simulink library "dspmathops"  (Simulink 6.0)
settings: Solver=ode45  SolverMode=SingleTasking  StartTime=0.0  StopTime=10.0  RelTol=1e-3
values from neighbouring files (symbols this model uses):
  D = D + B    [rebuffer_delay.m]
undefined symbols (not defined in the file or in its folder): dBval, fuzz_val, magnitude
libraries: dspsigattribs x2
settings Model: RequirementInfo=9  CovMetricSettings=d  ForwardingTableString=||__slOldName__||dspmathops/DSP Sum||__slNewName__||dspobslib/DSP Sum||__slOldName__||dspmathops/DSP Product||__slNewName__||dspobslib/DSP Product||__slOldName__||dspmathops/DSP Gain||__slNewName__||dspobslib/DSP Gain  Creator=don  LastModifiedBy=mlongfri  ExtModeAutoUpdateStatusClock=off  ProdHWDeviceType=Specified
settings DataIOCC: SignalLoggingName=logsOut
settings OptimizationCC: BooleanDataType=off
settings DebuggingCC: CheckExecutionContextPreStartOutputMsg=on  CheckExecutionContextRuntimeOutputMsg=on  SolverPrmCheckMsg=none
settings HardwareCC: ProdHWDeviceType=Specified  TargetUnknown=on
settings SFSimCC: SFSimApplyToAllLibs=on  SFSimBuildMode=Incremental

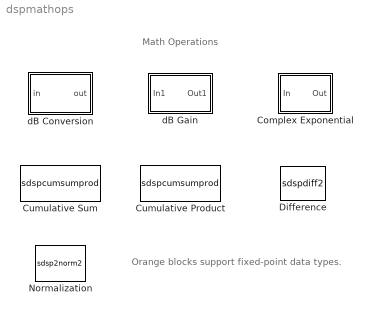
== system dspmathops ==
  note: Math Operations
  note: Orange blocks support fixed-point data types.
  Complex Exponential : Subsystem  PropExecContextAcrossSSBoundary=on
      mask Type: Complex Exponential
      mask Description:
      | Compute the complex exponential function of real inputs via
      | Euler's formula, y = cos(x)+jsin(x).
      mask Help: web(dspbhelp);
      mask Display: text(0.2, 0.55,'exp(jx)');
  Cumulative Product : S-Function  DialogController=dspDDGCreate  DialogControllerArgs=DataTag0  FunctionName=sdspcumsumprod  Parameters=dim,reset,fcn,dtInfo.interProdMode,dtInfo.interProdWordLength,dtInfo.interProdFracLength,dtInfo.prodOutputMode,dtInfo.prodOutputWordLength,dtInfo.prodOutputFracLength,dtInfo.accumMode,dtInfo.accumWordLength,dtInfo.accumFracLength,dtInfo.outputMode,dtInfo.outputWordLength,dtInfo.outputFracLength,dtInfo.roundingMode,dtInfo.overflowMode  mask(Cumulative Product){dim=Channels (running product), reset_popup=None, interProdMode=Same as input, interProdWordLength=16, interProdFracLength=15, prodOutputMode=Same as input, prodOutputWordLength=32, prodOutputFracLength=30, accumMode=Same as input, accumWordLength=32, accumFracLength=30, outputMode=Same as input, outputWordLength=16, outputFracLength=15, roundingMode=Floor, overflowMode=off, LockScale=off}
      mask prompts: dim "Multiply input along:"; reset_popup "Reset port:"; interProdMode "inter prod mode"; interProdWordLength "inter prod wl"; interProdFracLength "inter prod fl"; prodOutputMode "prod output mode"; prodOutputWordLength "prod output wl"; prodOutputFracLength "prod output fl"; accumMode "accum mode"; accumWordLength "accum wl"; accumFracLength "accum fl"; outputMode "output mode"; outputWordLength "output wl"; outputFracLength "output fl"; roundingMode "rm"; overflowMode "om"; LockScale "Lock scaling"
      mask help: Cumulative product of input matrix or input vector elements along the specified dimension: rows, columns, or channels. For 1-D and sample-based inputs, each element of the input matrix or vector is a channel. For frame-based inputs, each column of the input matrix or vector is a channel.
      mask init:
      | s = dspblkcumsumprod('icon');
      | reset=reset_popup-1;
      | fcn=1;
      | 
      | dtInfo = dspGetFixptDataTypeInfo(gcbh,271);
      settings: CopyFcn=dspfixptcopycallback
      mask Help: web(dspbhelp);
      mask StyleString: popup(Columns|Rows|Channels (running product)),popup(None|Rising edge|Falling edge|Either edge|Non-zero sample),popup(Same as input|Binary point scaling|Slope and bias scaling),edit,edit,popup(Same as input|Binary point scaling|Slope and bias scaling),edit,edit,popup(Same as product output|Same as input|Binary point scaling|Slope and bias scaling),edit,edit,popup(Same as product output|Same as input|Binary point scaling|Slope and bias scaling),edit,edit,popup(Floor|Nearest),checkbox,checkbox
      mask Display:
      | disp([s.str '\nProduct'])
      | port_label('input',s.i1,s.i1s);
      | port_label('input',s.i2,s.i2s);
  Cumulative Sum : S-Function  DialogController=dspDDGCreate  DialogControllerArgs=DataTag1  FunctionName=sdspcumsumprod  Parameters=dim,reset,fcn,-1,0,0,-1,0,0,dtInfo.accumMode,dtInfo.accumWordLength,dtInfo.accumFracLength,dtInfo.outputMode,dtInfo.outputWordLength,dtInfo.outputFracLength,dtInfo.roundingMode,dtInfo.overflowMode  mask(Cumulative Sum){dim=Channels (running sum), reset_popup=None, accumMode=Same as input, accumWordLength=32, accumFracLength=30, outputMode=Same as accumulator, outputWordLength=16, outputFracLength=15, roundingMode=Floor, overflowMode=off, LockScale=off}
      mask prompts: dim "Sum input along:"; reset_popup "Reset port:"; accumMode "accMode"; accumWordLength "accWL"; accumFracLength "accFL"; outputWordLength "outputWL"; outputFracLength "outputFL"; roundingMode "rm"; overflowMode "om"; LockScale "Lock scaling"
      mask help: Cumulative sum of input matrix or input vector elements along the specified dimension: rows, columns, or channels. For 1-D and sample-based inputs, each element of the input matrix or vector is a channel. For frame-based inputs, each column of the input matrix or vector is a channel.
      mask init:
      | s = dspblkcumsumprod('icon');
      | reset=reset_popup-1;
      | fcn=0;
      | 
      | dtInfo = dspGetFixptDataTypeInfo(gcbh,7);
      settings: CopyFcn=dspfixptcopycallback
      mask Help: web(dspbhelp);
      mask StyleString: popup(Columns|Rows|Channels (running sum)),popup(None|Rising edge|Falling edge|Either edge|Non-zero sample),popup(Same as input|Binary point scaling|Slope and bias scaling),edit,edit,popup(Same as accumulator|Same as input|Binary point scaling|Slope and bias scaling),edit,edit,popup(Floor|Nearest),checkbox,checkbox
      mask Display:
      | disp([s.str '\nSum'])
      | port_label('input',s.i1,s.i1s);
      | port_label('input',s.i2,s.i2s);
  Difference : S-Function  DialogController=dspDDGCreate  DialogControllerArgs=DataTag2  FunctionName=sdspdiff2  Parameters=dim,dtInfo.accumMode,dtInfo.accumWordLength,dtInfo.accumFracLength,dtInfo.outputMode,dtInfo.outputWordLength,dtInfo.outputFracLength,dtInfo.roundingMode,dtInfo.overflowMode  mask(Difference){dim=Columns, additionalParams=off, allowOverrides=on, outputMode=Same as accumulator, outputWordLength=16, outputFracLength=15, accumMode=Inherit via internal rule, accumWordLength=32, accumFracLength=30, roundingMode=Floor, overflowMode=off, LockScale=off}
      mask prompts: dim "Difference along:"; additionalParams "------- Show additional parameters -------"; allowOverrides "Allow overrides from DSP Fixed-Point Attributes blocks"; outputMode "Fixed-point output attributes:"; outputWordLength "Output word length:"; outputFracLength "Output fraction length:"; accumMode "Fixed-point accumulator attributes:"; accumWordLength "Accumulator word length:"; accumFracLength "Accumulator fraction length:"; roundingMode "Round integer calculations toward:"; overflowMode "Saturate on integer overflow"; LockScale "Lock scaling"
      mask help: Difference between adjacent input elements. For oriented inputs, difference along the specified dimension.
      mask init:
      | if (dim==1), str='Row\nDiff';
      | else str='Column\nDiff';
      | end
      | dtInfo = dspGetFixptDataTypeInfo(gcbh,7);
      settings: CopyFcn=dspfixptcopycallback
      mask Help: web(dspbhelp);
      mask StyleString: popup(Rows|Columns),checkbox,checkbox,popup(Same as accumulator|Same as input|Binary point scaling|Slope and bias scaling|User-defined),edit,edit,popup(Inherit via internal rule|Same as input|Binary point scaling|Slope and bias scaling|User-defined),edit,edit,popup(Floor|Nearest),checkbox,checkbox
      mask Display: disp(str)
  Normalization : S-Function  DialogController=dspDDGCreate  DialogControllerArgs=DataTag3  FunctionName=sdsp2norm2  Parameters=Bias,NormType,dtInfo.prodOutputMode,dtInfo.prodOutputWordLength,dtInfo.prodOutputFracLength,dtInfo.accumMode,dtInfo.accumWordLength,dtInfo.accumFracLength,dtInfo.outputMode,dtInfo.outputWordLength,dtInfo.outputFracLength,dtInfo.roundingMode,dtInfo.overflowMode  mask(Normalization){NormType=Squared 2-norm, Bias=1e-10, additionalParams=off, allowOverrides=on, outputMode=Same as product output, outputWordLength=32, outputFracLength=32, accumMode=Same as product output, accumWordLength=32, accumFracLength=30, prodOutputMode=Same as input, prodOutputWordLength=32, prodOutputFracLength=32, roundingMode=Floor, overflowMode=off, LockScale=off}
      mask prompts: NormType "Norm:"; Bias "Normalization bias:"; additionalParams "--------------- Show additional parameters ---------------"; allowOverrides "Allow overrides from DSP Attributes blocks"; outputMode "Fixed-point output attributes:"; outputWordLength "Output word length:"; outputFracLength "Output fraction length:"; accumMode "Fixed-point accumulator attributes"; accumWordLength "Accumulator word length:"; accumFracLength "Accumulator fraction length:"; prodOutputMode "Fixed-point product output attributes:"; prodOutputWordLength "Product output word length:"; prodOutputFracLength "Product output fraction length:"; roundingMode "Round integer calculations toward:"; overflowMode "Saturate on integer overflow"; LockScale "Lock scaling"
      mask help: Normalize each input element by the vector 2-norm, sqrt(u'u)+b, or by the squared 2-norm, u'u+b, where b is a bias used to protect against divide-by-zero. Normalization is performed along the columns for matrix inputs.
      mask init:
      | x = [0 NaN 100 NaN 20 80 NaN 30 30 NaN 36 36 NaN 58 58 NaN 64 64];
      | y = [0 NaN 100 NaN 60 60 NaN 9 43 NaN 9 43 NaN 9 43 NaN 9 43];
      | if NormType==1, sqr_txt = ' '; else sqr_txt = '2'; end
      | dtInfo = dspGetFixptDataTypeInfo(gcbh,15);
      settings: CopyFcn=dspfixptcopycallback
      mask Help: web(dspbhelp);
      mask StyleString: popup(2-norm|Squared 2-norm),edit,checkbox,checkbox,popup(Same as product output|Same as accumulator|Same as input|Binary point scaling|Slope and bias scaling),edit,edit,popup(Same as product output|Same as input|Binary point scaling|Slope and bias scaling),edit,edit,popup(Same as input|Binary point scaling|Slope and bias scaling),edit,edit,popup(Floor|Nearest),checkbox,checkbox
      mask Display:
      | plot(x,y)
      | text(44,80,'u'); text(44,25,'u'); text(72,39,sqr_txt)
  dB Conversion : Subsystem  PropExecContextAcrossSSBoundary=on  mask(dB Conversion){dBtype=dB, intype=Amplitude, R=1, fuzz=off}
      mask prompts: dBtype "Convert to:"; intype "Input signal:"; R "Load resistance (ohms):"; fuzz "Add  eps to input to protect against  "log(0) = -inf""
      mask help: Convert input of Watts or Volts to decibels. Voltage inputs are first converted to power relative to the specified load resistance, where P = (V^2)/R. When converting to dBm, the power is scaled to units of mWatts.
      mask init:
      | [str fuzz_val dBval] = dspblkdb2('init');
      | dspblkdb2('checkparam');
      | dspblkdb2('update');
      mask Help: web(dspbhelp);
      mask StyleString: popup(dB|dBm),popup(Power|Amplitude),edit,checkbox
      mask CallbackString: dspblkdb2|dspblkdb2||
      mask Display: disp(str)
  dB Gain : Subsystem  PropExecContextAcrossSSBoundary=on  mask(dB Gain){dB=-40, intype=Amplitude}
      mask prompts: dB "Gain, dB:"; intype "Input signal:"
      mask help: Apply a gain specified in dB.
      mask init:
      | if isempty(dB)
      |   dB = 0; g = 0;
      |   s  = ['dB Gain'];
      | else
      |   g=10.^(dB/(10*intype));
      |   if (isscalar(dB))
      |     s = sprintf('%g dB\n(%g)',dB,g);
      |   else
      |     s = ['dB Gain'];
      |   end
      | end
      settings: CopyFcn=dspfixptcopycallback
      mask Help: web(dspbhelp);
      mask StyleString: edit,popup(Power|Amplitude)
      mask Display: fprintf(s)

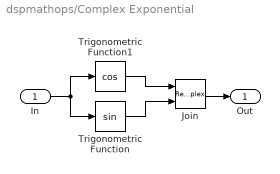
== system dspmathops/Complex Exponential ==
  In : Inport  LatchInput=off
  Join : RealImagToComplex
  Trigonometric Function : Trigonometry
  Trigonometric Function1 : Trigonometry  Operator=cos
  Out : Outport
  wires:
  Trigonometric Function1/1 -> Join/1
  Trigonometric Function/1 -> Join/2
  Join/1 -> Out/1
  In/1 -> Trigonometric Function1/1, Trigonometric Function/1

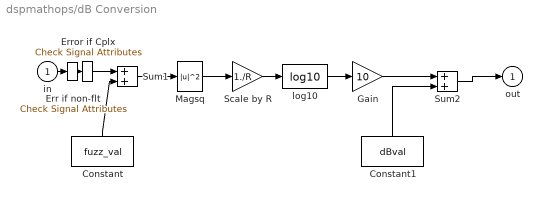
== system dspmathops/dB Conversion ==
  in : Inport  LatchInput=off
  Constant : Constant  Orientation=up  Value=fuzz_val
  Constant1 : Constant  Orientation=up  Value=dBval
  Err if non-flt : dspsigattribs/Check Signal Attributes  SigAttribCheckMethod=Does not match attributes exactly  Complexity=Ignore  Frame=Ignore  DimsCheckMethod=Ignore  Dimensions=1-D  DatatypeCheckMethod=Is...  DatatypeGeneral=Floating-point  DtypeFloatSpecific=Any floating-point  DtypeFixedSpecific=Any fixed-point  DtypeIntSpecific=Any integer  SampleMode=Ignore
  Error if Cplx : dspsigattribs/Check Signal Attributes  SigAttribCheckMethod=Matches attributes exactly  Complexity=Complex  Frame=Ignore  DimsCheckMethod=Ignore  Dimensions=1-D  DatatypeCheckMethod=Ignore  DatatypeGeneral=Boolean  DtypeFloatSpecific=Any floating-point  DtypeFixedSpecific=Any fixed-point  DtypeIntSpecific=Any integer  SampleMode=Ignore
  Gain : Gain  Gain=10  SaturateOnIntegerOverflow=on
  Magsq : Math  Operator=magnitude^2  SaturateOnIntegerOverflow=on
  Scale by R : Gain  Gain=1./R  SaturateOnIntegerOverflow=on
  Sum1 : Sum  SaturateOnIntegerOverflow=on  InputSameDT=on
  Sum2 : Sum  SaturateOnIntegerOverflow=on  InputSameDT=on
  log10 : Math  Operator=log10  SaturateOnIntegerOverflow=on
  out : Outport  InitialOutput=0
  wires:
  Constant1/1 -> Sum2/2
  Sum2/1 -> out/1
  Gain/1 -> Sum2/1
  Constant/1 -> Sum1/2
  Sum1/1 -> Magsq/1
  Error if Cplx/1 -> Sum1/1
  in/1 -> Err if non-flt/1
  Err if non-flt/1 -> Error if Cplx/1
  Scale by R/1 -> log10/1
  Magsq/1 -> Scale by R/1
  log10/1 -> Gain/1

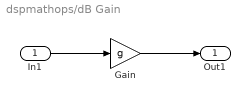
== system dspmathops/dB Gain ==
  In1 : Inport  LatchInput=off
  Gain : Gain  Gain=g
  Out1 : Outport
  wires:
  In1/1 -> Gain/1
  Gain/1 -> Out1/1
